simulink model "LQRFINALEMODEL"  (R2021b)
settings: Solver=VariableStepAuto  StartTime=0.0  StopTime=380  RelTol=1e-3
values from neighbouring files (symbols this model uses):
  a = a/2    (= 0.1)    [DOF6Script.m]
  b = b/2    (= -0.25)    [DOF6Script.m]
  c = c/2    (= 1000)    [DOF6Script.m]
  d = d/2    (= 1000)    [DOF6Script.m]
undefined symbols (not defined in the file or in its folder): A, Continuous, K_LQR, Time
libraries: simulink x7, cstblocks x3, ctrlSharedLib x2
settings Model: Creator=gugli  LastModifiedBy=alela

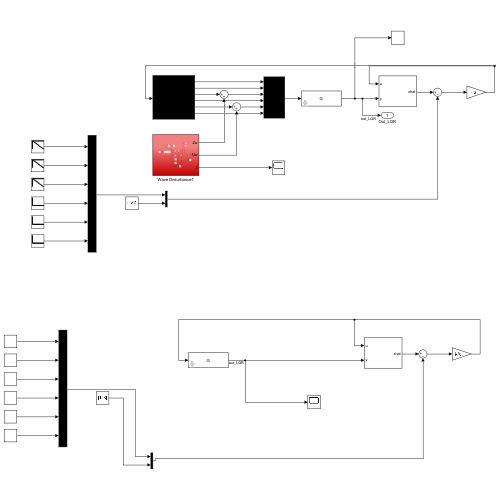
[thumbnail: Simulink's stored preview of the top-level diagram]
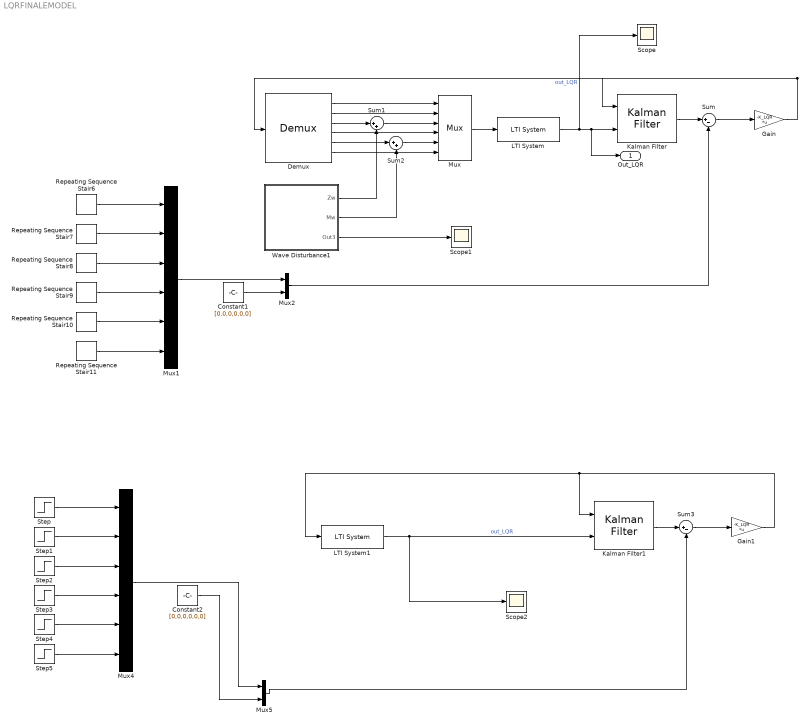
== system LQRFINALEMODEL ==
  Constant1 : Constant  Value=[0,0,0,0,0,0]
  Constant2 : Constant  Value=[0,0,0,0,0,0]
  Demux : Demux  Outputs=6
  Gain : Gain  Gain=-K_LQR  Multiplication=Matrix(K*u)
  Gain1 : Gain  Gain=-K_LQR  Multiplication=Matrix(K*u)
  Kalman Filter : ctrlSharedLib/Kalman Filter  TimeDomain=Continuous-Time  UseCurrentEstimator=on  ModelSource=LTI State-Space Variable  ModelSourceVariable=linsys1  A=A  B=1  C=1  D=0  NumberOfStates=1  NumberOfInputs=1  NumberOfOutputs=1  InitialEstimateSource=Dialog  X0=0  P0=10  UseK=off  UseGH=off  NumberOfProcessNoiseInputs=1  G=1  TimeInvariantG=on  H=0  TimeInvariantH=on  Q=0.05  TimeInvariantQ=on  R=1  TimeInvariantR=on  N=0  TimeInvariantN=on  AddInputPort=on  AddEnablePort=off  OutputEstimatedY=off  OutputP=off  Ts=-1
  Kalman Filter1 : ctrlSharedLib/Kalman Filter  TimeDomain=Continuous-Time  UseCurrentEstimator=on  ModelSource=LTI State-Space Variable  ModelSourceVariable=linsys1  A=A  B=1  C=1  D=0  NumberOfStates=1  NumberOfInputs=1  NumberOfOutputs=1  InitialEstimateSource=Dialog  X0=0  P0=10  UseK=off  UseGH=off  NumberOfProcessNoiseInputs=1  G=1  TimeInvariantG=on  H=0  TimeInvariantH=on  Q=0.05  TimeInvariantQ=on  R=1  TimeInvariantR=on  N=0  TimeInvariantN=on  AddInputPort=on  AddEnablePort=off  OutputEstimatedY=off  OutputP=off  Ts=-1
  LTI System : cstblocks/LTI System  sys=G  IC=[]
  LTI System1 : cstblocks/LTI System  sys=G  IC=[]
  Mux : Mux  Inputs=6
  Mux1 : Mux  Inputs=6
  Mux2 : Mux  Inputs=2
  Mux4 : Mux  Inputs=6
  Mux5 : Mux  Inputs=2
  Repeating Sequence Stair10 : simulink/Sources/Repeating Sequence Stair  OutValues=pich_trajectory  tsamp=sample_time  OutMin=[]  OutMax=[]  OutDataTypeStr=double  OutputDataTypeScalingMode=double  OutDataType=fixdt(0,8)  ConRadixGroup=Best Precision: Vector-wise  OutScaling=2^-12
  Repeating Sequence Stair11 : simulink/Sources/Repeating Sequence Stair  OutValues=yaw_trajectory  tsamp=sample_time  OutMin=[]  OutMax=[]  OutDataTypeStr=double  OutputDataTypeScalingMode=double  OutDataType=fixdt(0,8)  ConRadixGroup=Best Precision: Vector-wise  OutScaling=2^-12
  Repeating Sequence Stair6 : simulink/Sources/Repeating Sequence Stair  OutValues=x_trajectory  tsamp=sample_time  OutMin=[]  OutMax=[]  OutDataTypeStr=double  OutputDataTypeScalingMode=double  OutDataType=fixdt(0,8)  ConRadixGroup=Best Precision: Vector-wise  OutScaling=2^-12
  Repeating Sequence Stair7 : simulink/Sources/Repeating Sequence Stair  OutValues=y_trajectory  tsamp=sample_time  OutMin=[]  OutMax=[]  OutDataTypeStr=double  OutputDataTypeScalingMode=double  OutDataType=fixdt(0,8)  ConRadixGroup=Best Precision: Vector-wise  OutScaling=2^-12
  Repeating Sequence Stair8 : simulink/Sources/Repeating Sequence Stair  OutValues=z_trajectory  tsamp=sample_time  OutMin=[]  OutMax=[]  OutDataTypeStr=double  OutputDataTypeScalingMode=double  OutDataType=fixdt(0,8)  ConRadixGroup=Best Precision: Vector-wise  OutScaling=2^-12
  Repeating Sequence Stair9 : simulink/Sources/Repeating Sequence Stair  OutValues=roll_trajectory  tsamp=sample_time  OutMin=[]  OutMax=[]  OutDataTypeStr=double  OutputDataTypeScalingMode=double  OutDataType=fixdt(0,8)  ConRadixGroup=Best Precision: Vector-wise  OutScaling=2^-12
  Scope : Scope
  Scope1 : Scope
  Scope2 : Scope
  Step{,1..5} (6 alike) : Step  SampleTime=0
  Sum : Sum  Inputs=|+-
  Sum1 : Sum  Inputs=|++
  Sum2 : Sum  Inputs=|++
  Sum3 : Sum  Inputs=|+-
  Wave Disturbance1 : Subsystem
  Out_LQR : Outport
  wires:
  Gain/1 -> Demux/1, Kalman Filter/1
  LTI System/1 -> Scope/1, Out_LQR/1, Kalman Filter/2  "out_LQR"
  Kalman Filter/1 -> Sum/1
  Sum/1 -> Gain/1
  Mux1/1 -> Mux2/1
  Repeating Sequence Stair9/1 -> Mux1/4
  Repeating Sequence Stair8/1 -> Mux1/3
  Repeating Sequence Stair6/1 -> Mux1/1
  Repeating Sequence Stair10/1 -> Mux1/5
  Repeating Sequence Stair11/1 -> Mux1/6
  Repeating Sequence Stair7/1 -> Mux1/2
  Constant1/1 -> Mux2/2
  Mux2/1 -> Sum/2
  Mux/1 -> LTI System/1
  Demux/1 -> Mux/1
  Demux/2 -> Mux/2
  Demux/4 -> Mux/4
  Demux/6 -> Mux/6
  Demux/3 -> Sum1/1
  Sum1/1 -> Mux/3
  Demux/5 -> Sum2/1
  Sum2/1 -> Mux/5
  Wave Disturbance1/1(Zw) -> Sum1/2
  Wave Disturbance1/2(Mw) -> Sum2/2
  Wave Disturbance1/3(Out3) -> Scope1/1
  Gain1/1 -> LTI System1/1, Kalman Filter1/1
  LTI System1/1 -> Kalman Filter1/2, Scope2/1  "out_LQR"
  Sum3/1 -> Gain1/1
  Constant2/1 -> Mux5/2
  Kalman Filter1/1 -> Sum3/1
  Step4/1 -> Mux4/5
  Step2/1 -> Mux4/3
  Mux5/1 -> Sum3/2
  Step5/1 -> Mux4/6
  Step1/1 -> Mux4/2
  Step/1 -> Mux4/1
  Mux4/1 -> Mux5/1
  Step3/1 -> Mux4/4

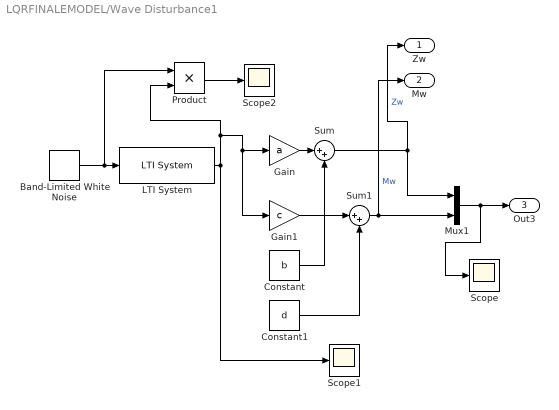
== system LQRFINALEMODEL/Wave Disturbance1 ==
  Band-Limited White Noise : simulink/Sources/Band-Limited White Noise  Cov=[0.1]  Ts=0.01  seed=[23341]
  Constant : Constant  Value=b
  Constant1 : Constant  Value=d
  Gain : Gain  Gain=a
  Gain1 : Gain  Gain=c
  LTI System : cstblocks/LTI System  sys=G4  IC=[]
  Mux1 : Mux  Inputs=2
  Product : Product
  Scope : Scope
  Scope1 : Scope
  Scope2 : Scope
  Sum : Sum  Inputs=|++
  Sum1 : Sum  Inputs=|++
  Zw : Outport
  Mw : Outport  Port=2
  Out3 : Outport  Port=3
  wires:
  Sum/1 -> Zw/1, Mux1/1  "Zw"
  Gain/1 -> Sum/1
  Gain1/1 -> Sum1/1
  Constant/1 -> Sum/2
  Band-Limited White Noise/1 -> Product/1, LTI System/1
  Sum1/1 -> Mux1/2, Mw/1  "Mw"
  Constant1/1 -> Sum1/2
  Mux1/1 -> Scope/1, Out3/1
  LTI System/1 -> Scope1/1, Product/2, Gain1/1, Gain/1
  Product/1 -> Scope2/1
